simulink model "Steer_ff"  (R2023a)
settings: Solver=ode4  StartTime=0.0  StopTime=5  FixedStep=0.001  RelTol=1e-3
libraries: simulink x1
settings Model: Creator=KBISWAS  LastModifiedBy=KBISWAS

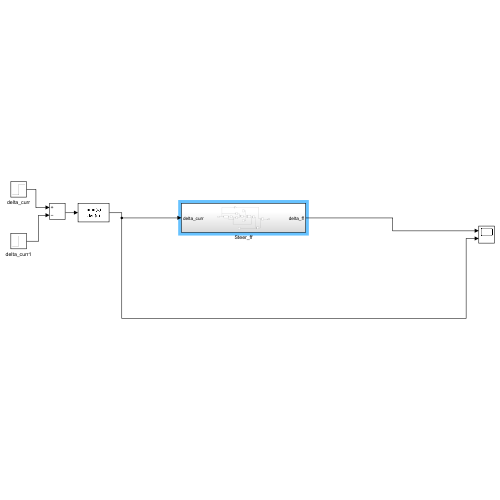
[thumbnail: Simulink's stored preview of the top-level diagram]
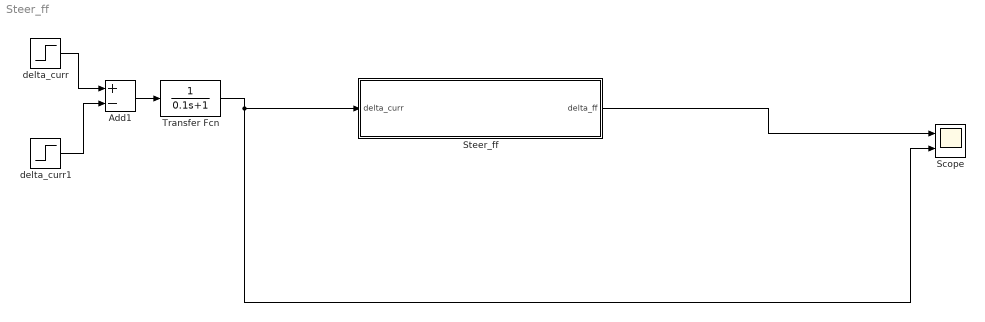
== system Steer_ff ==
  Add1 : Sum  Inputs=+-
  Scope : Scope  NumInputPorts=2
  Steer_ff : Subsystem
  Transfer Fcn : TransferFcn  Denominator=[0.1 1]
  delta_curr : Step  After=10  SampleTime=0
  delta_curr1 : Step  Time=3  After=10  SampleTime=0
  wires:
  Transfer Fcn/1 -> Steer_ff/1(delta_curr), Scope/2
  delta_curr/1 -> Add1/1
  delta_curr1/1 -> Add1/2
  Add1/1 -> Transfer Fcn/1
  Steer_ff/1(delta_ff) -> Scope/1

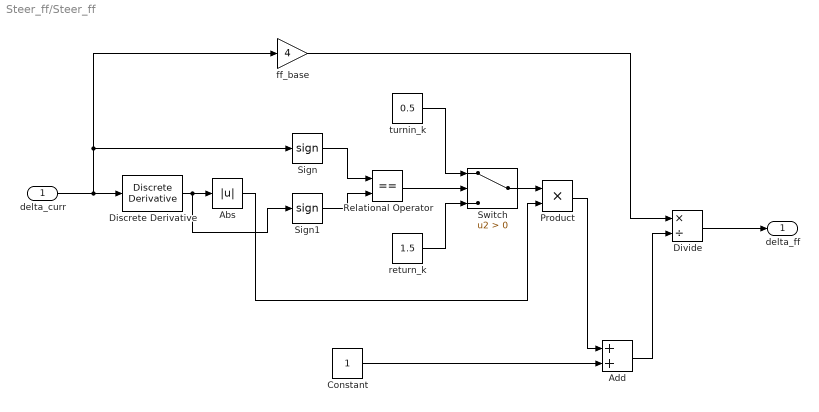
== system Steer_ff/Steer_ff ==
  delta_curr : Inport
  Abs : Abs  SaturateOnIntegerOverflow=off
  Add : Sum
  Constant : Constant
  Discrete Derivative : simulink/Discrete/Discrete Derivative  gainval=1.0  ICPrevScaledInput=0.0  OutMin=[]  OutMax=[]  OutDataType=fixdt(1, 16)  OutScaling=2^-10  DoSatur=off
  Divide : Product  Inputs=*/
  Product : Product
  Relational Operator : RelationalOperator  Operator===  OutDataTypeStr=boolean  RndMeth=Simplest  InputSameDT=off
  Sign : Signum
  Sign1 : Signum
  Switch : Switch  Criteria=u2 > Threshold  SaturateOnIntegerOverflow=off  InputSameDT=off
  ff_base : Gain  Gain=4
  return_k : Constant  Value=1.5
  turnin_k : Constant  Value=0.5
  delta_ff : Outport
  wires:
  ff_base/1 -> Divide/1
  return_k/1 -> Switch/3
  Switch/1 -> Product/1
  Product/1 -> Add/1
  Sign/1 -> Relational Operator/1
  delta_curr/1 -> Discrete Derivative/1, ff_base/1, Sign/1
  Relational Operator/1 -> Switch/2
  Add/1 -> Divide/2
  Discrete Derivative/1 -> Sign1/1, Abs/1
  Abs/1 -> Product/2
  Constant/1 -> Add/2
  Sign1/1 -> Relational Operator/2
  Divide/1 -> delta_ff/1
  turnin_k/1 -> Switch/1
